simulink model "quadFly"  (R2019b)
settings: Solver=ode4  StartTime=0.0  StopTime=inf  FixedStep=0.001  RelTol=1e-3
InitFcn:
  | Init_control;
values from neighbouring files (symbols this model uses):
  Kd_RP_AgngleRate = 0.005    [Init_control.m]    (also in quadFly.sldd)
  Kd_YAW_AngleRate = 0.05    [Init_control.m]    (also in quadFly.sldd)
  Ki_RP_AgngleRate = 0.01    [Init_control.m]    (also in quadFly.sldd)
  Ki_YAW_AngleRate = 0.8    [Init_control.m]    (also in quadFly.sldd)
  Kp_RP_AgngleRate = 0.55    [Init_control.m]    (also in quadFly.sldd)
  Kp_RP_ANGLE = 6.5    [Init_control.m]    (also in quadFly.sldd)
  Kp_YAW_AngleRate = 3.2    [Init_control.m]    (also in quadFly.sldd)
  MAX_CONTROL_ANGLE_RATE_Y = 90    [Init_control.m]    (also in quadFly.sldd = 90.0)
  ModelInit_RPM = 0.0    [quadFly.sldd]
  ModelParam_envAltitude = -41.5260009765625    [quadFly.sldd]
  ModelParam_GlobalNoiseGainSwitch = 1.0    [quadFly.sldd]
  ModelParam_GPSLatLong = 40.1540302 116.2593683    [quadFly.sldd]
  ModelParam_motorCr = 1148.0    [quadFly.sldd]
  ModelParam_motorJm = 0.0001287    [quadFly.sldd]
  ModelParam_motorMinThr = 0.05    [quadFly.sldd]
  ModelParam_motorT = 0.02    [quadFly.sldd]
  ModelParam_motorWb = -141.4    [quadFly.sldd]
  ModelParam_rotorCm = 1.779E-7    [quadFly.sldd]
  ModelParam_rotorCt = 1.105E-5    [quadFly.sldd]
  ModelParam_uavCCm = 0.01 0.01 0.0055    [quadFly.sldd]
  ModelParam_uavCd = 0.073    [quadFly.sldd]
  ModelParam_uavDearo = 0.12    [quadFly.sldd]
  ModelParam_uavJ = 0.0211 0.0 0.0 0.0 0.0219 0.0 0.0 0.0 0.0366    [quadFly.sldd]
  ModelParam_uavMass = 1.4    [quadFly.sldd]
  ModelParam_uavR = 0.225    [quadFly.sldd]
  ModelParam_uavType = 3    [quadFly.sldd]
undefined symbols (not defined in the file or in its folder): DWORK0, DWORK1, DWORK10, DWORK11, DWORK12, DWORK13, DWORK14, DWORK15, DWORK2, DWORK3, DWORK4, DWORK5, DWORK6, DWORK7, DWORK8, DWORK9, earthRadius, KiPitchAttitude, KiRollAttitude, Receive, Send
libraries: simulink x15, ctrl_ADRC_angular_rate x4, aerolibfltsims x3, ctrl_ADRC_TD x2, shared6dof x1, aerolibanimutils x1
(part 4 of 4)

== matlab function quadFly/ADRC_Controller /pwm_out1 ==
  data: Roll input; M1 output; Pitch input; Yaw input; Thrust input; M2 output; M3 output; M4 output
function [M1, M2, M3, M4] = motor_mixer(Roll, Pitch, Yaw, Thrust)

idle_PWM = 1000;

% Quad XROLL （根据QP里面的叉字形结构的文字）
% M1 = ((Pitch+ Yaw)+Thrust-Roll) * 1000 + idle_PWM;
 %M2 = ((Pitch - Yaw)+Thrust+Roll) * 1000 + idle_PWM;
 %M3 = ((Roll +Yaw) + Thrust-Pitch) * 1000 + idle_PWM;
 %M4 = ((-Roll - Pitch-Yaw) + Thrust) * 1000 + idle_PWM;
% M5 = 1000;
% M6 = 1000;
% M7 = 1000;
% M8 = 1000;
%qp上实际的输出
M1 = (Thrust+Pitch-Roll+Yaw)*1000  + idle_PWM;
M2 = (Thrust-Pitch +Roll+Yaw)*1000 + idle_PWM;
M3 = (Thrust+Roll+Pitch-Yaw)*1000  + idle_PWM;
M4 = (Thrust-Roll- Pitch -Yaw)*1000 + idle_PWM;
% Quad +
 %M1 = ((Pitch - Yaw) * Thrust / 2 + Thrust) * 1000 + idle_PWM;
 %M2 = ((-Roll + Yaw) * Thrust / 2 + Thrust) * 1000 + idle_PWM;
% M3 = ((-Pitch - Yaw) * Thrust / 2 + Thrust) * 1000 + idle_PWM;
 %M4 = ((Roll + Yaw) * Thrust / 2 + Thrust) * 1000 + idle_PWM;
% M5 = 1000;
% M6 = 1000;
% M7 = 1000;
% M8 = 1000;

% Hex X
% M1 = ((Pitch + Roll / 2 - Yaw) * Thrust / 2 + Thrust) * 1000 + idle_PWM;
% M2 = ((Pitch - Roll / 2 + Yaw) * Thrust / 2 + Thrust) * 1000 + idle_PWM;
% M3 = ((-Roll - Yaw) * Thrust / 2 + Thrust) * 1000 + idle_PWM;
% M4 = ((-Pitch - Roll / 2 + Yaw) * Thrust / 2 + Thrust) * 1000 + idle_PWM;
% M5 = ((-Pitch + Roll / 2 - Yaw) * Thrust / 2 + Thrust) * 1000 + idle_PWM;
% M6 = ((Roll + Yaw) * Thrust / 2 + Thrust) * 1000 + idle_PWM;
% M7 = 1000;
% M8 = 1000;

% Hex X (From Adam)
%M1 = uint16(single(((-Roll - Yaw) * Thrust / 3 + Thrust) * single(1000))) + idle_PWM;
%M2 = uint16(single(((Roll + Yaw) * Thrust / 3 + Thrust) * single(1000))) + idle_PWM;
%M3 = uint16(single(((Pitch + (Roll / 2) - Yaw) * Thrust / 3 + Thrust) * single(1000))) + idle_PWM;
%M4 = uint16(single(((-Pitch - (Roll / 2) + Yaw) * Thrust / 3 + Thrust) * single(1000))) + idle_PWM;
%M5 = uint16(single(((Pitch - (Roll / 2) + Yaw) * Thrust / 3 + Thrust) * single(1000))) + idle_PWM;
%M6 = uint16(single(((-Pitch + (Roll / 2) - Yaw) * Thrust / 3 + Thrust) * single(1000))) + idle_PWM;

% Hex X (Version 2)
% Roll/Yaw
% M1 = ((-Roll - Yaw) * Thrust / 2 + Thrust) * 1000 + idle_PWM;
% M2 = ((Roll + Yaw) * Thrust / 2 + Thrust) * 1000 + idle_PWM;
% % + Pitch/Roll
% M6 = ((Pitch + Roll / 2 - Yaw) * Thrust / 2 + Thrust) * 1000 + idle_PWM;
% M4 = ((Pitch - Roll / 2 + Yaw) * Thrust / 2 + Thrust) * 1000 + idle_PWM;
% % - Pitch/Roll
% M5 = ((-Pitch - Roll / 2 + Yaw) * Thrust / 2 + Thrust) * 1000 + idle_PWM;
% M3 = ((-Pitch + Roll / 2 - Yaw) * Thrust / 2 + Thrust) * 1000 + idle_PWM;

== matlab function quadFly/Control System1/InputConditioning/MATLAB Function3 ==
  data: u input; y output
function y = fcn(u)
%将遥控输入的范围控制在1100~1900，同时设置一个死区，死区大小为±deadZone
RCMin = 1100;
RCMax = 1900;
deadZoneRate = 0.05;
deadZone = deadZoneRate*(RCMax-RCMin);
%限幅
if(u < RCMin)
    u = RCMin;
elseif(u > RCMax)
    u = RCMax;
end
%死区
 if(u > 1500+deadZone)
    y = u;
 elseif(u < 1500-deadZone)
     y = u;
 else
     y = 1500;
 end
     
 end
